simulink model "ContinSoftStart_55kWt_done_v20_discrete"  (R2014a)
settings: Solver=ode23tb  StartTime=0.0  StopTime=5  MaxStep=1e-3  RelTol=1e-6
values from neighbouring files (symbols this model uses):
  f = 50    [M_ContinSoftStarter_55kWt.m]
  J = 0.0059    [AM_4A100S2Y3.m]    (also in M_ContinSoftStarter_55kWt.m = 0.25)
  Kpr = 4.7    [M_ContinSoftStarter_55kWt.m]
  L1e = L1_    [AM_4A100S2Y3.m]    (also in M_ContinSoftStarter_55kWt.m = 0.0014)
  L1sig = x1sig/Wsn    [AM_4A100S2Y3.m]    (also in M_ContinSoftStarter_55kWt.m = 0.000638)
  L2sig = x2sig/Wsn    [AM_4A100S2Y3.m]    (also in M_ContinSoftStarter_55kWt.m = 0.000821)
  P2n = 4000    [AM_4A100S2Y3.m]
  ph_deg = [0 -120 120]    [M_ContinSoftStarter_55kWt.m]
  PIREG_K_prop = L1e/(To1*Kpr)    (= 0.0297872340426)    [M_ContinSoftStarter_55kWt.m]
  PIREG_T_integ = 1/(r1e/(To1*Kpr))    (= 0.489073881374)    [M_ContinSoftStarter_55kWt.m]
  r1 = tR1*Zb    [AM_4A100S2Y3.m]    (also in M_ContinSoftStarter_55kWt.m = 0.0567)
  r1e = r1 + r2*k2^2    [AM_4A100S2Y3.m]    (also in M_ContinSoftStarter_55kWt.m = 0.0961)
  r2 = tR2*Zb    [AM_4A100S2Y3.m]    (also in M_ContinSoftStarter_55kWt.m = 0.0409)
  To1 = 0.01    [M_ContinSoftStarter_55kWt.m]
  Ts = 1e-6    (= 1e-06)    [M_ContinSoftStarter_55kWt.m]
  Vm = Vrms*sqrt(2)    [M_ContinSoftStarter_55kWt.m]
undefined symbols (not defined in the file or in its folder): DiscIntNeverNeededParam
libraries: powerlib x13, simulink x3
settings Model: Creator=NPT  LastModifiedBy=user

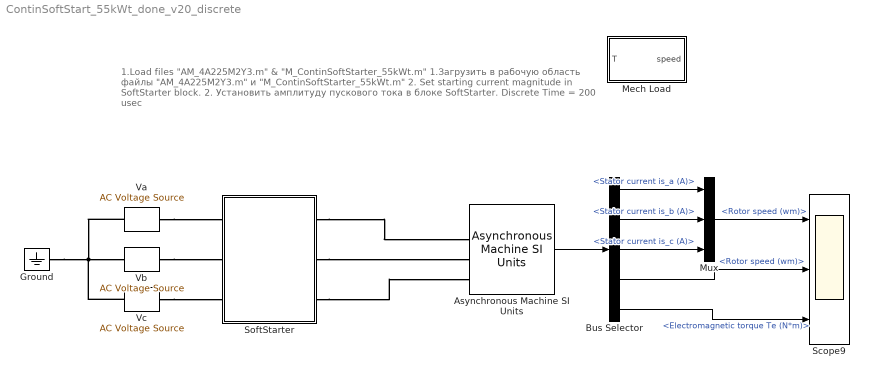
== system ContinSoftStart_55kWt_done_v20_discrete ==
  note: 1.Load files "AM_4A225M2Y3.m" & "M_ContinSoftStarter_55kWt.m"
      | 1.Загрузить в рабочую область файлы "AM_4A225M2Y3.m" и "M_ContinSoftStarter_55kWt.m"
      |
      | 2. Set starting current magnitude in SoftStarter block.
      | 2. Установить амплитуду пускового тока в блоке SoftStarter.
      |
      |
      | Discrete Time = 200 usec
  Asynchronous Machine SI Units : powerlib/Machines/Asynchronous Machine SI Units  PresetModel=No  MechanicalLoad=Torque Tm  ShowDetailedParameters=on  RotorType=Squirrel-cage  ReferenceFrame=Rotor  Units=SI  MeasurementBus=off  NominalParameters=[P2n 380 50]  Stator=[r1 L1sig]  Rotor=[r2 L2sig]  Cage1=[ 0.022 0.226/377]  Cage2=[ 0.022 0.226/377]  Lm=L0  Mechanical=[J 0 1]  PolePairs=2  InitialConditions=[1 0 0 0 0 0 0 0]  SimulateSaturation=off  Saturation=[14.03593122, 27.81365428, 53.79336849, 72.68890987, 97.98006896, 148.6815601, 215.7428561, 302.9841135, 420.4778367 ; 230, 322, 414, 460, 506, 552, 598, 644, 690]  LoadFlowParameters=1492000  TsPowergui=0  TsBlock=-1  IterativeModel=Trapezoidal non iterative  Pmec=10000
  Bus Selector : BusSelector  OutputSignals=Stator measurements.Stator current is_a (A),Stator measurements.Stator current is_b (A),Stator measurements.Stator current is_c (A),Mechanical.Rotor speed (wm),Mechanical.Electromagnetic torque Te (N*m)
  Ground : powerlib/Elements/Ground  LConnTagsString=a
  Mech Load : Subsystem
  Mux : Mux  Inputs=3
  Scope9 : Scope  NumInputPorts=3
      settings: TimeRange=0.0566164604626143  YMin=-17.5~56~0.7  YMax=17.5~80~1.85
  SoftStarter : Subsystem  mask{Istart=8}
      mask prompts: Istart "I_start, A"
  Va : powerlib/Electrical Sources/AC Voltage Source  Amplitude=Vm  Phase=ph_deg(1)  Frequency=f  SampleTime=-1  Measurements=None
  Vb : powerlib/Electrical Sources/AC Voltage Source  Amplitude=Vm  Phase=ph_deg(2)  Frequency=f  SampleTime=-1  Measurements=None
  Vc : powerlib/Electrical Sources/AC Voltage Source  Amplitude=Vm  Phase=ph_deg(3)  Frequency=f  SampleTime=-1  Measurements=None
  wires:
  Asynchronous Machine SI Units/1 -> Bus Selector/1
  Bus Selector/3 -> Mux/3  "<Stator current is_c (A)>"
  Bus Selector/2 -> Mux/2  "<Stator current is_b (A)>"
  Bus Selector/1 -> Mux/1  "<Stator current is_a (A)>"
  Bus Selector/4 -> Scope9/2  "<Rotor speed (wm)>"
  Bus Selector/5 -> Scope9/3  "<Electromagnetic torque Te (N*m)>"
  Mux/1 -> Scope9/1  "<Rotor speed (wm)>"
  connections:
  Ground/LConn1 -- Vb/LConn1 -- Va/LConn1 -- Vc/LConn1
  Vc/RConn1 -- SoftStarter/LConn3
  Vb/RConn1 -- SoftStarter/LConn2
  Va/RConn1 -- SoftStarter/LConn1
  SoftStarter/RConn2 -- Asynchronous Machine SI Units/LConn2
  SoftStarter/RConn3 -- Asynchronous Machine SI Units/LConn3
  SoftStarter/RConn1 -- Asynchronous Machine SI Units/LConn1

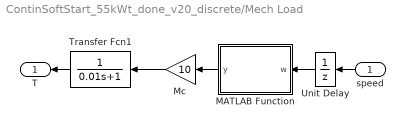
== system ContinSoftStart_55kWt_done_v20_discrete/Mech Load ==
  speed : Inport
  MATLAB Function : MATLAB Function  TreatAsAtomicUnit=on
  Mc : Gain  Gain=10
  Transfer Fcn1 : TransferFcn  Denominator=[0.01 1]
  Unit Delay : UnitDelay  SampleTime=-1
  T : Outport
  wires:
  MATLAB Function/1(y) -> Mc/1
  Unit Delay/1 -> MATLAB Function/1(w)
  Mc/1 -> Transfer Fcn1/1
  Transfer Fcn1/1 -> T/1
  speed/1 -> Unit Delay/1

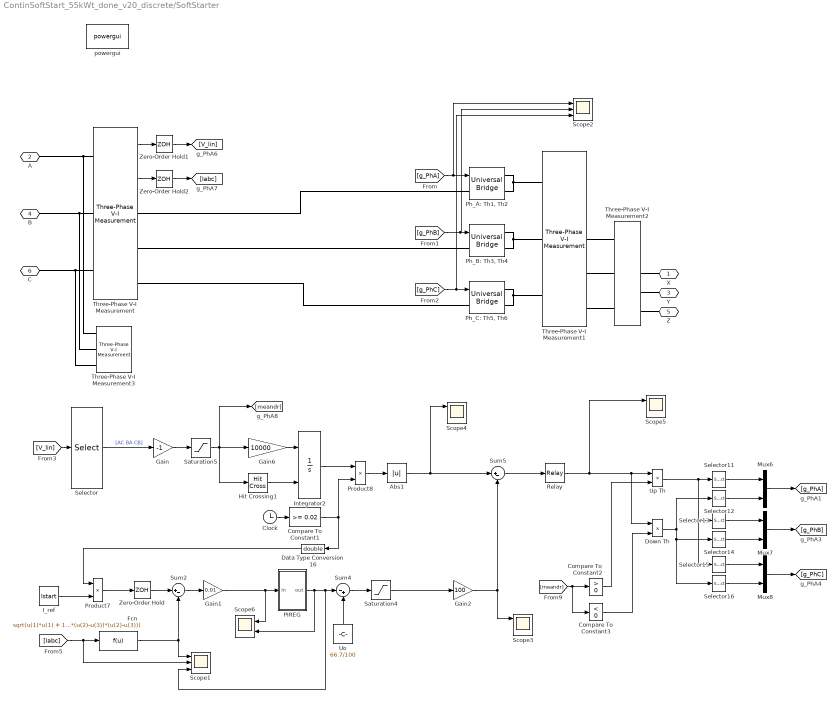
== system ContinSoftStart_55kWt_done_v20_discrete/SoftStarter ==
  Abs1 : Abs
  Clock : Clock
  Compare To Constant1 : simulink/Logic and Bit Operations/Compare To Constant  relop=>=  const=0.02  OutDataTypeStr=boolean
  Compare To Constant2 : simulink/Logic and Bit Operations/Compare To Constant  relop=>  const=0  OutDataTypeStr=uint8
  Compare To Constant3 : simulink/Logic and Bit Operations/Compare To Constant  relop=<  const=0  OutDataTypeStr=uint8
  Data Type Conversion16 : DataTypeConversion  OutDataTypeStr=double
  Down Th : Product
  Fcn : Fcn  Expr=sqrt(u(1)*u(1) + 1/3*(u(2)-u(3))*(u(2)-u(3)))
  Gain : Gain  Gain=-1
  Gain1 : Gain  Gain=0.01
  Gain2 : Gain  Gain=100
  Gain6 : Gain  Gain=10000
  Hit Crossing1 : HitCross
  I_ref : Constant  Value=Istart
  Integrator2 : Integrator  ExternalReset=either  LimitOutput=on  UpperSaturationLimit=100  LowerSaturationLimit=-100
  Mux6 : Mux  Inputs=2
  Mux7 : Mux  Inputs=2
  Mux8 : Mux  Inputs=2
  PIREG : Subsystem
  "Ph_A: Th1, Th2" : powerlib/Power Electronics/Universal Bridge  Arms=1  SnubberResistance=1e5  SnubberCapacitance=inf  Device=Thyristors  Ron=1e-3  Lon=0  ForwardVoltages="[  0  0  ]"  ForwardVoltage=0  GTOparameters=[ 10e-6 , 20e-6 ]  IGBTparameters=[ 1e-6 , 2e-6 ]  Measurements=None  Measurements_2=None  converterType=Rectifier
  "Ph_B: Th3, Th4 " : powerlib/Power Electronics/Universal Bridge  Arms=1  SnubberResistance=1e5  SnubberCapacitance=inf  Device=Thyristors  Ron=1e-3  Lon=0  ForwardVoltages="[  0  0  ]"  ForwardVoltage=0  GTOparameters=[ 10e-6 , 20e-6 ]  IGBTparameters=[ 1e-6 , 2e-6 ]  Measurements=None  Measurements_2=None  converterType=Rectifier
  "Ph_C: Th5, Th6" : powerlib/Power Electronics/Universal Bridge  Arms=1  SnubberResistance=1e5  SnubberCapacitance=inf  Device=Thyristors  Ron=1e-3  Lon=0  ForwardVoltages="[  0  0  ]"  ForwardVoltage=0  GTOparameters=[ 10e-6 , 20e-6 ]  IGBTparameters=[ 1e-6 , 2e-6 ]  Measurements=None  Measurements_2=None  converterType=Rectifier
  Product7 : Product
  Product8 : Product  OutDataTypeStr=double
  Relay : Relay
  Saturation4 : Saturate  UpperLimit=66.7/100  LowerLimit=2.8/100
  Saturation5 : Saturate  UpperLimit=1  LowerLimit=-1
  Scope{1..5} (5 alike) : Scope  NumInputPorts=3
      Scope1 settings: TimeRange=0.0566164604626143  YMin=0~-35~11.8  YMax=40~35~13.2
      Scope2 settings: TimeRange=0.0566164604626143  YMin=-0.007~0~-5  YMax=0.007~1~5  SaveName=ScopeData2
      Scope3 settings: TimeRange=0.0566164604626143  YMin=0.0062~-1~-1  YMax=0.008~1~1  SaveName=ScopeData3
      Scope4 settings: TimeRange=0.0566164604626143  YMin=0.0062~-1~-1  YMax=0.008~1~1  SaveName=ScopeData4
      Scope5 settings: TimeRange=0.0566164604626143  YMin=0.0062~-1~-1  YMax=0.008~1~1  SaveName=ScopeData5
  Scope6 : Scope  NumInputPorts=2
      settings: TimeRange=0.0566164604626143  YMin=0.076~0.63365  YMax=0.084~0.70035  SaveName=ScopeData6
  Selector : Selector  InputPortWidth=3  Indices=[3 1 2]
  Selector11 : Selector  InputPortWidth=3  Indices=[1]
  Selector12 : Selector  InputPortWidth=3  Indices=[1]
  Selector13 : Selector  InputPortWidth=3  Indices=[2]
  Selector14 : Selector  InputPortWidth=3  Indices=[2]
  Selector15 : Selector  InputPortWidth=3  Indices=[3]
  Selector16 : Selector  InputPortWidth=3  Indices=[3]
  Sum2 : Sum  Inputs=|+-
  Sum4 : Sum  Inputs=|-+
  Sum5 : Sum  Inputs=|+-
  Three-Phase V-I Measurement : powerlib/Measurements/Three-Phase V-I Measurement  VoltageMeasurement=phase-to-phase  SetLabelV=off  LabelV=Vabc  Vpu=off  VpuLL=off  CurrentMeasurement=yes  SetLabelI=off  LabelI=Iabc  Ipu=off  Pbase=100e6  Vbase=500e3  OutputType=Complex  PhasorSimulation=off  PSBequivalent=0
  Three-Phase V-I Measurement1 : powerlib/Measurements/Three-Phase V-I Measurement  VoltageMeasurement=phase-to-ground  SetLabelV=off  LabelV=Vabc  Vpu=off  VpuLL=off  CurrentMeasurement=yes  SetLabelI=off  LabelI=Iabc  Ipu=off  Pbase=100e6  Vbase=500e3  OutputType=Complex  PhasorSimulation=off  PSBequivalent=0
  Three-Phase V-I Measurement2 : powerlib/Measurements/Three-Phase V-I Measurement  VoltageMeasurement=phase-to-ground  SetLabelV=off  LabelV=Vabc  Vpu=off  VpuLL=off  CurrentMeasurement=yes  SetLabelI=off  LabelI=Iabc  Ipu=off  Pbase=100e6  Vbase=500e3  OutputType=Complex  PhasorSimulation=off  PSBequivalent=0
  Three-Phase V-I Measurement3 : powerlib/Measurements/Three-Phase V-I Measurement  VoltageMeasurement=phase-to-ground  SetLabelV=off  LabelV=Vabc  Vpu=off  VpuLL=off  CurrentMeasurement=yes  SetLabelI=off  LabelI=Iabc  Ipu=off  Pbase=100e6  Vbase=500e3  OutputType=Complex  PhasorSimulation=off  PSBequivalent=0
  Uo : Constant  Value=66.7/100
  Up Th : Product
  Zero-Order Hold : ZeroOrderHold  SampleTime=2e-4
  Zero-Order Hold1 : ZeroOrderHold  SampleTime=2e-4
  Zero-Order Hold2 : ZeroOrderHold  SampleTime=2e-4
  powergui : powerlib/powergui  Priority=1  SimulationMode=Continuous  SolverType=Tustin  SampleTime=Ts  frequency=60  SPID=off  DisableSnubberDevices=off  DisableRonSwitches=off  DisableVfSwitches=off  SwTol=0  Interpol=off  DisplayEquations=off  Ts=0  methode=off  frequencyindice=50  Pbase=100e6  ErrMax=1e-4  Iterations=50  UnitsV=kV  UnitsW=MW  FunctionMessages=off  echomessages=off  HookPort=off  EnableUseOfTLC=off  x0status=zero  RestoreLinks=warning  ResistiveCurrentMeasurement=off  Frange=[0:2:500]  Ylog=off  Xlog=on  ShowGrid=off  save=off  variable=ZData  structure=0  ZoomFFT=off  StartTime=0.0  cycles=1  DisplayStyle=1  fundamental=60  FreqAxis=off  MaxFrequency=1000  frequencyindicesteady=1  RmsSteady=1  display=off
  X : PMIOPort  Port=1  Side=Right
  A : PMIOPort  Port=2  Side=Left
  Y : PMIOPort  Port=3  Side=Right
  B : PMIOPort  Port=4  Side=Left
  Z : PMIOPort  Port=5  Side=Right
  C : PMIOPort  Port=6  Side=Left
  wires:
  Three-Phase V-I Measurement/2 -> Zero-Order Hold2/1
  Three-Phase V-I Measurement/1 -> Zero-Order Hold1/1
  [V_lin] -> Selector/1
  Selector/1 -> Gain/1  "[AC BA CB]"
  Sum4/1 -> Saturation4/1
  [g_PhA] -> Scope2/1, "Ph_A: Th1, Th2"/1
  [g_PhB] -> Scope2/2, "Ph_B: Th3, Th4 "/1
  [g_PhC] -> Scope2/3, "Ph_C: Th5, Th6"/1
  [Iabc] -> Scope1/2, Fcn/1
  Fcn/1 -> Sum2/2, Scope1/1
  I_ref/1 -> Product7/2
  Uo/1 -> Sum4/2
  Product7/1 -> Zero-Order Hold/1
  Gain/1 -> Saturation5/1
  Gain6/1 -> Integrator2/1
  Saturation5/1 -> [meandr], Hit Crossing1/1, Gain6/1
  Hit Crossing1/1 -> Integrator2/2
  Clock/1 -> Compare To Constant1/1
  Integrator2/1 -> Product8/1
  Compare To Constant1/1 -> Data Type Conversion16/1, Product8/2
  Product8/1 -> Abs1/1
  Saturation4/1 -> Gain2/1
  Sum5/1 -> Relay/1
  [meandr] -> Compare To Constant3/1, Compare To Constant2/1
  Relay/1 -> Scope5/1, Down Th/1, Up Th/1
  Compare To Constant2/1 -> Up Th/2
  Compare To Constant3/1 -> Down Th/2
  Up Th/1 -> Selector13/1, Selector15/1, Selector11/1
  Selector11/1 -> Mux6/1
  Down Th/1 -> Selector14/1, Selector16/1, Selector12/1
  Selector12/1 -> Mux6/2
  Selector14/1 -> Mux7/2
  Selector13/1 -> Mux7/1
  Selector16/1 -> Mux8/2
  Selector15/1 -> Mux8/1
  Data Type Conversion16/1 -> Product7/1
  Mux6/1 -> [g_PhA]
  Mux7/1 -> [g_PhB]
  Mux8/1 -> [g_PhC]
  Zero-Order Hold/1 -> Sum2/1
  Zero-Order Hold1/1 -> [V_lin]
  Zero-Order Hold2/1 -> [Iabc]
  Abs1/1 -> Scope4/1, Sum5/1
  PIREG/1(out) -> Scope6/2, Sum4/1, Scope1/3
  Sum2/1 -> Gain1/1
  Gain1/1 -> Scope6/1, PIREG/1(in)
  Gain2/1 -> Scope3/1, Sum5/2
  connections:
  C/RConn1 -- Three-Phase V-I Measurement3/LConn3 -- Three-Phase V-I Measurement/LConn3
  B/RConn1 -- Three-Phase V-I Measurement3/LConn2 -- Three-Phase V-I Measurement/LConn2
  A/RConn1 -- Three-Phase V-I Measurement3/LConn1 -- Three-Phase V-I Measurement/LConn1
  Three-Phase V-I Measurement/RConn3 -- "Ph_C: Th5, Th6"/LConn1
  "Ph_A: Th1, Th2"/LConn1 -- Three-Phase V-I Measurement/RConn1
  "Ph_C: Th5, Th6"/RConn1 -- "Ph_C: Th5, Th6"/RConn2 -- Three-Phase V-I Measurement1/LConn3
  "Ph_B: Th3, Th4 "/RConn1 -- "Ph_B: Th3, Th4 "/RConn2 -- Three-Phase V-I Measurement1/LConn2
  "Ph_A: Th1, Th2"/RConn1 -- Three-Phase V-I Measurement1/LConn1 -- "Ph_A: Th1, Th2"/RConn2
  "Ph_B: Th3, Th4 "/LConn1 -- Three-Phase V-I Measurement/RConn2
  Three-Phase V-I Measurement1/RConn2 -- Three-Phase V-I Measurement2/LConn2
  Three-Phase V-I Measurement1/RConn1 -- Three-Phase V-I Measurement2/LConn1
  Three-Phase V-I Measurement1/RConn3 -- Three-Phase V-I Measurement2/LConn3
  Three-Phase V-I Measurement2/RConn1 -- X/RConn1
  Three-Phase V-I Measurement2/RConn2 -- Y/RConn1
  Three-Phase V-I Measurement2/RConn3 -- Z/RConn1

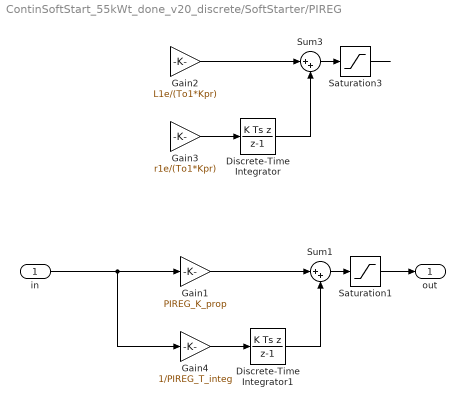
== system ContinSoftStart_55kWt_done_v20_discrete/SoftStarter/PIREG ==
  in : Inport
  Discrete-Time Integrator : DiscreteIntegrator  IntegratorMethod=Integration: Backward Euler  SampleTime=2e-4  LimitOutput=on  UpperSaturationLimit=66.7/100  LowerSaturationLimit=0  ICPrevOutput=DiscIntNeverNeededParam  ICPrevScaledInput=DiscIntNeverNeededParam
  Discrete-Time Integrator1 : DiscreteIntegrator  IntegratorMethod=Integration: Backward Euler  SampleTime=2e-4  LimitOutput=on  UpperSaturationLimit=66.7/100  LowerSaturationLimit=0  ICPrevOutput=DiscIntNeverNeededParam  ICPrevScaledInput=DiscIntNeverNeededParam
  Gain1 : Gain  Gain=PIREG_K_prop
  Gain2 : Gain  Gain=L1e/(To1*Kpr)
  Gain3 : Gain  Gain=r1e/(To1*Kpr)
  Gain4 : Gain  Gain=1/PIREG_T_integ
  Saturation1 : Saturate  UpperLimit=66.7/100  LowerLimit=0
  Saturation3 : Saturate  UpperLimit=66.7/100  LowerLimit=0
  Sum1 : Sum  Inputs=|++
  Sum3 : Sum  Inputs=|++
  out : Outport
  wires:
  ? -> Gain3/1, Gain2/1
  Gain3/1 -> Discrete-Time Integrator/1
  Gain2/1 -> Sum3/1
  Discrete-Time Integrator/1 -> Sum3/2
  Sum3/1 -> Saturation3/1
  Saturation3/1 -> ?
  in/1 -> Gain1/1, Gain4/1
  Gain4/1 -> Discrete-Time Integrator1/1
  Gain1/1 -> Sum1/1
  Discrete-Time Integrator1/1 -> Sum1/2
  Sum1/1 -> Saturation1/1
  Saturation1/1 -> out/1

== matlab function ContinSoftStart_55kWt_done_v20_discrete/Mech Load/MATLAB Function ==
  data: w input; y output
function y = fcn(w)
%#codegen

if w > 0.01
    temp = 1;
elseif w < -0.01
    temp = -1;
else
    temp = 0;  
end

y = temp;
